simulink model "DynamicsAaa"  (R2017a)
settings: Solver=VariableStepAuto  StartTime=0.0  StopTime=200  RelTol=1e-3
(part 1 of 8)
settings Model: Creator=Aaa  LastModifiedBy=Aaa

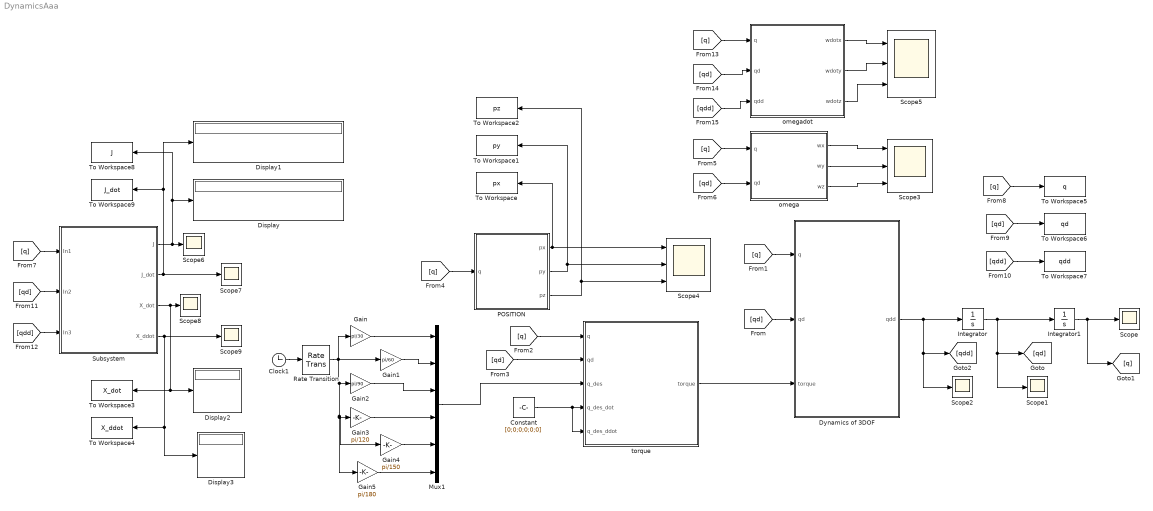
== system DynamicsAaa ==
  Clock1 : Clock
  Constant : Constant  Value=[0;0;0;0;0;0]
  Display{,1..3} (4 alike) : Display
  Dynamics of 3DOF : MATLAB Function  TreatAsAtomicUnit=on
  Gain : Gain  Gain=pi/30
  Gain1 : Gain  Gain=pi/60
  Gain2 : Gain  Gain=pi/90
  Gain3 : Gain  Gain=pi/120
  Gain4 : Gain  Gain=pi/150
  Gain5 : Gain  Gain=pi/180
  Integrator : Integrator  InitialCondition=[0;0;0;0;0;0]
  Integrator1 : Integrator  InitialCondition=[1;1;1;1;1;1]
  Mux1 : Mux  Inputs=6
  POSITION : MATLAB Function  TreatAsAtomicUnit=on
  Rate Transition : RateTransition  OutPortSampleTime=10
  Scope{,1..2,6..9} (7 alike) : Scope
  Scope3 : Scope  NumInputPorts=3
  Scope4 : Scope  NumInputPorts=3
  Scope5 : Scope  NumInputPorts=3
  Subsystem : Subsystem
  To Workspace : ToWorkspace  VariableName=px  SampleTime=-1
  To Workspace1 : ToWorkspace  VariableName=py  SampleTime=-1
  To Workspace2 : ToWorkspace  VariableName=pz  SampleTime=-1
  To Workspace3 : ToWorkspace  VariableName=X_dot  SampleTime=-1
  To Workspace4 : ToWorkspace  VariableName=X_ddot  SampleTime=-1
  To Workspace5 : ToWorkspace  VariableName=q  SampleTime=-1
  To Workspace6 : ToWorkspace  VariableName=qd  SampleTime=-1
  To Workspace7 : ToWorkspace  VariableName=qdd  SampleTime=-1
  To Workspace8 : ToWorkspace  VariableName=J  SampleTime=-1
  To Workspace9 : ToWorkspace  VariableName=J_dot  SampleTime=-1
  omega : MATLAB Function  TreatAsAtomicUnit=on
  omegadot : MATLAB Function  TreatAsAtomicUnit=on
  torque : MATLAB Function  TreatAsAtomicUnit=on
  wires:
  Dynamics of 3DOF/1(qdd) -> [qdd], Scope2/1, Integrator/1
  Integrator1/1 -> [q], Scope/1
  Integrator/1 -> Integrator1/1, Scope1/1, [qd]
  [q] -> To Workspace5/1
  torque/1(torque) -> Dynamics of 3DOF/3(torque)
  [q] -> torque/1(q)
  [qdd] -> To Workspace7/1
  [qd] -> To Workspace6/1
  [qd] -> Dynamics of 3DOF/2(qd)
  Constant/1 -> torque/5(q_des_ddot), torque/4(q_des_dot)
  [qd] -> torque/2(qd)
  [q] -> Dynamics of 3DOF/1(q)
  POSITION/1(px) -> To Workspace/1, Scope4/1
  [q] -> POSITION/1(q)
  POSITION/3(pz) -> To Workspace2/1, Scope4/3
  POSITION/2(py) -> To Workspace1/1, Scope4/2
  [q] -> omega/1(q)
  [qd] -> omega/2(qd)
  omega/1(wx) -> Scope3/1
  omega/2(wy) -> Scope3/2
  omega/3(wz) -> Scope3/3
  [qd] -> Subsystem/2(In2)
  Subsystem/2(J_dot) -> To Workspace9/1, Display1/1, Scope7/1
  Subsystem/3(X_dot) -> To Workspace3/1, Display2/1, Scope8/1
  Subsystem/4(X_ddot) -> Display3/1, To Workspace4/1, Scope9/1
  [qdd] -> Subsystem/3(In3)
  Subsystem/1(J) -> To Workspace8/1, Display/1, Scope6/1
  [q] -> Subsystem/1(In1)
  Rate Transition/1 -> Gain1/1, Gain5/1, Gain3/1, Gain4/1, Gain2/1, Gain/1
  Clock1/1 -> Rate Transition/1
  Gain2/1 -> Mux1/3
  Gain1/1 -> Mux1/2
  Gain3/1 -> Mux1/4
  Gain5/1 -> Mux1/6
  Gain4/1 -> Mux1/5
  Mux1/1 -> torque/3(q_des)
  Gain/1 -> Mux1/1
  omegadot/1(wdotx) -> Scope5/1
  [qd] -> omegadot/2(qd)
  [q] -> omegadot/1(q)
  omegadot/2(wdoty) -> Scope5/2
  omegadot/3(wdotz) -> Scope5/3
  [qdd] -> omegadot/3(qdd)

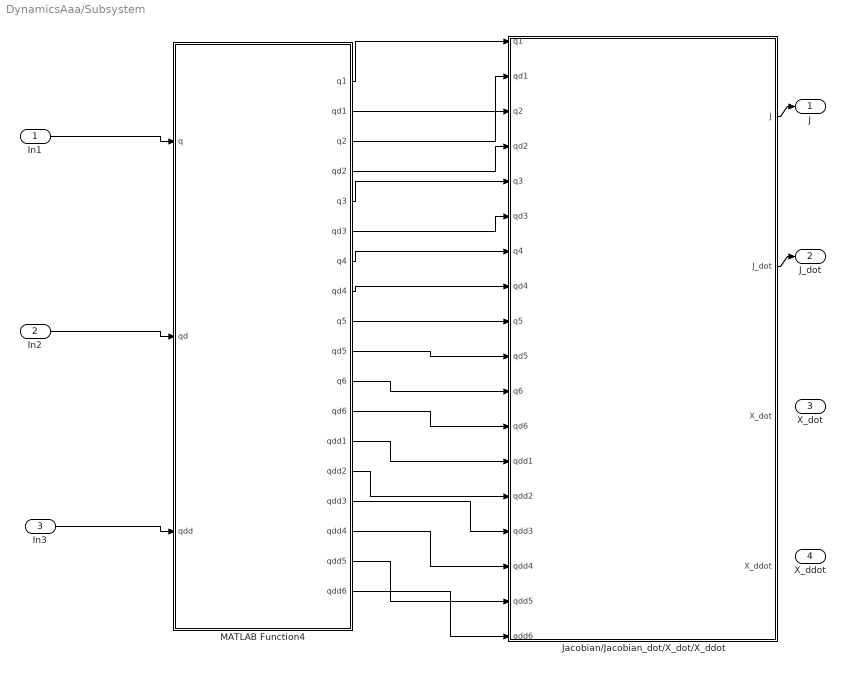
== system DynamicsAaa/Subsystem ==
  In1 : Inport
  In2 : Inport  Port=2
  In3 : Inport  Port=3
  Jacobian/Jacobian_dot/X_dot/X_ddot : MATLAB Function  TreatAsAtomicUnit=on
  MATLAB Function4 : MATLAB Function  TreatAsAtomicUnit=on
  J : Outport
  J_dot : Outport  Port=2
  X_dot : Outport  Port=3
  X_ddot : Outport  Port=4
  wires:
  In2/1 -> MATLAB Function4/2(qd)
  In3/1 -> MATLAB Function4/3(qdd)
  In1/1 -> MATLAB Function4/1(q)
  MATLAB Function4/3(q2) -> Jacobian/Jacobian_dot/X_dot/X_ddot/3(q2)
  MATLAB Function4/8(qd4) -> Jacobian/Jacobian_dot/X_dot/X_ddot/8(qd4)
  MATLAB Function4/4(qd2) -> Jacobian/Jacobian_dot/X_dot/X_ddot/4(qd2)
  MATLAB Function4/9(q5) -> Jacobian/Jacobian_dot/X_dot/X_ddot/9(q5)
  MATLAB Function4/2(qd1) -> Jacobian/Jacobian_dot/X_dot/X_ddot/2(qd1)
  MATLAB Function4/1(q1) -> Jacobian/Jacobian_dot/X_dot/X_ddot/1(q1)
  MATLAB Function4/5(q3) -> Jacobian/Jacobian_dot/X_dot/X_ddot/5(q3)
  MATLAB Function4/6(qd3) -> Jacobian/Jacobian_dot/X_dot/X_ddot/6(qd3)
  MATLAB Function4/7(q4) -> Jacobian/Jacobian_dot/X_dot/X_ddot/7(q4)
  Jacobian/Jacobian_dot/X_dot/X_ddot/1(J) -> J/1
  Jacobian/Jacobian_dot/X_dot/X_ddot/2(J_dot) -> J_dot/1
  ? -> X_dot/1
  ? -> X_ddot/1
  MATLAB Function4/10(qd5) -> Jacobian/Jacobian_dot/X_dot/X_ddot/10(qd5)
  MATLAB Function4/11(q6) -> Jacobian/Jacobian_dot/X_dot/X_ddot/11(q6)
  MATLAB Function4/12(qd6) -> Jacobian/Jacobian_dot/X_dot/X_ddot/12(qd6)
  MATLAB Function4/13(qdd1) -> Jacobian/Jacobian_dot/X_dot/X_ddot/13(qdd1)
  MATLAB Function4/14(qdd2) -> Jacobian/Jacobian_dot/X_dot/X_ddot/14(qdd2)
  MATLAB Function4/16(qdd4) -> Jacobian/Jacobian_dot/X_dot/X_ddot/16(qdd4)
  MATLAB Function4/15(qdd3) -> Jacobian/Jacobian_dot/X_dot/X_ddot/15(qdd3)
  MATLAB Function4/17(qdd5) -> Jacobian/Jacobian_dot/X_dot/X_ddot/17(qdd5)
  MATLAB Function4/18(qdd6) -> Jacobian/Jacobian_dot/X_dot/X_ddot/18(qdd6)
